simulink model "Task_3"  (R2023b)
settings: Solver=VariableStepAuto  StartTime=0.0  StopTime=10.0  RelTol=1e-3
libraries: simulink_extras x1
settings Model: Creator=danish  LastModifiedBy=danish

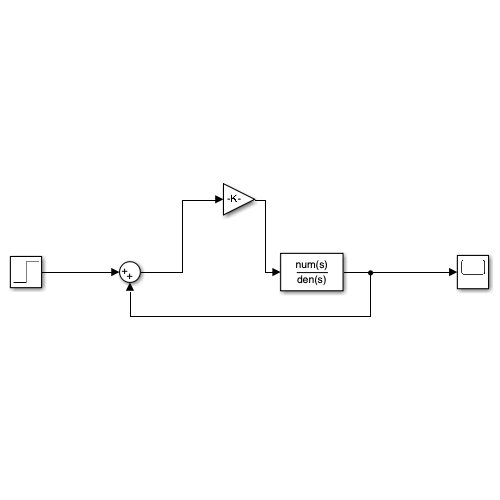
[thumbnail: Simulink's stored preview of the top-level diagram]
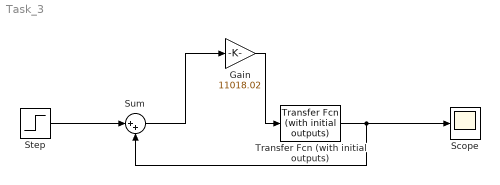
== system Task_3 ==
  Gain : Gain  Gain=11018.02
  Scope : Scope
  Step : Step  SampleTime=0
  Sum : Sum  Inputs=|++
  Transfer Fcn (with initial outputs) : simulink_extras/Additional Linear/Transfer Fcn (with initial outputs)  N=[1100 6611 66]  D=[1 130 3229 23480 58000 ]  Y0=.5  U0=0
  wires:
  Sum/1 -> Gain/1
  Step/1 -> Sum/1
  Gain/1 -> Transfer Fcn (with initial outputs)/1
  Transfer Fcn (with initial outputs)/1 -> Scope/1, Sum/2
